simulink model "nuri3s_dob__model_free"  (R2024b)
settings: Solver=VariableStepAuto  StartTime=0.0  StopTime=5  RelTol=1e-3
undefined symbols (not defined in the file): q_goal_rad, q_start
libraries: robotmaniplib x1, robotcorelib x1, simulink_extras x1
settings Model: Creator=변재형  LastModifiedBy=변재형

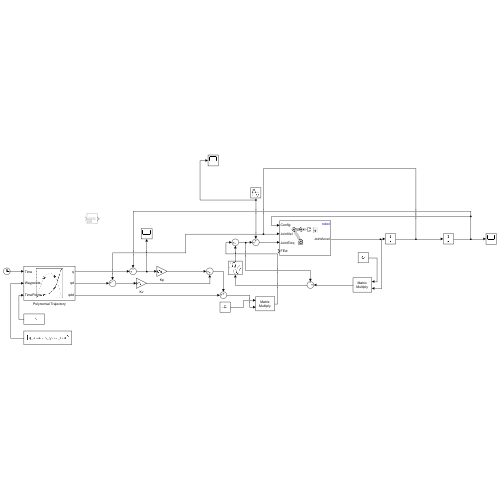
[thumbnail: Simulink's stored preview of the top-level diagram]
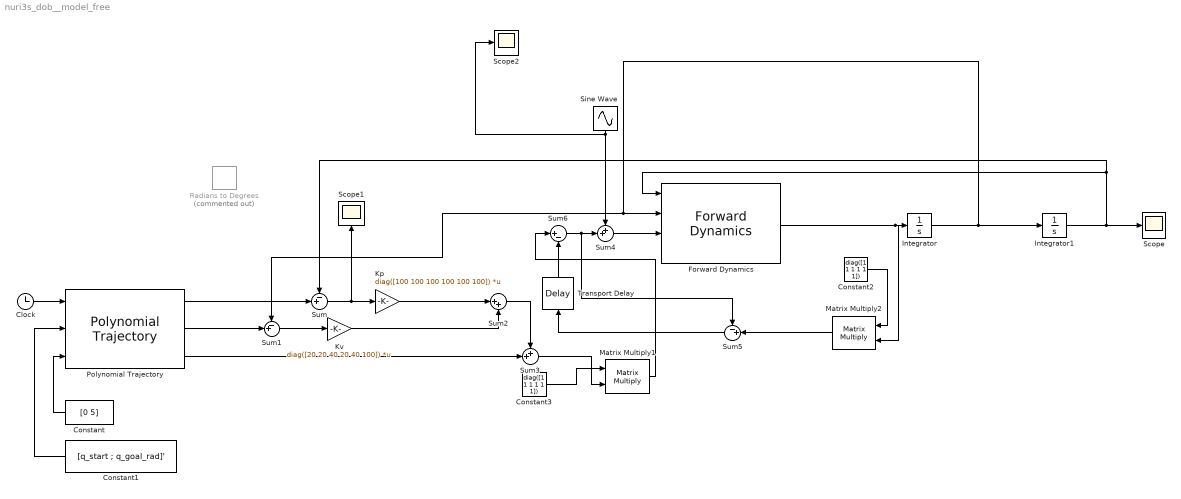
== system nuri3s_dob__model_free ==
  Clock : Clock
  Constant : Constant  Value=[0 5]
  Constant1 : Constant  Value=[q_start ; q_goal_rad]'
  Constant2 : Constant  Value=diag([1 1 1 1 1 1])
  Constant3 : Constant  Value=diag([1 1 1 1 1 1])
  Forward Dynamics : robotmaniplib/Forward Dynamics  RigidBodyTree=robot  SimulateUsing=Interpreted execution
  Integrator : Integrator
  Integrator1 : Integrator
  Kp : Gain  Gain=diag([100 100 100 100 100 100])  Multiplication=Matrix(K*u)
  Kv : Gain  Gain=diag([20 20 40 20 40 100])  Multiplication=Matrix(K*u)
  Matrix Multiply1 : Product  Multiplication=Matrix(*)
  Matrix Multiply2 : Product  Multiplication=Matrix(*)
  Polynomial Trajectory : robotcorelib/Polynomial Trajectory  WaypointSource=External  Waypoints=[ 0, 2, 1, 5, 0; -1, 3, 1, 4, 4 ]  TimePoints=[ 0, 1, 2, 3, 4 ]  TimeInterval=[ 1, 4 ]  Method=Quintic Polynomial  ParameterSource=Internal  VelocityBoundaryCondition=zeros( 6, 2 )  AccelerationBoundaryCondition=zeros( 6, 2 )  SimulateUsing=Interpreted execution
  Radians to Degrees : simulink_extras/Transformations/Radians to Degrees  Commented=on
  Scope : Scope
  Scope1 : Scope
  Scope2 : Scope
  Sine Wave : Sin  Amplitude=0.1  Frequency=10  SampleTime=0
  Sum : Sum  Inputs=-+|
  Sum1 : Sum  Inputs=-+|
  Sum2 : Sum  Inputs=|++
  Sum3 : Sum  Inputs=++|
  Sum4 : Sum  Inputs=++|
  Sum5 : Sum  Inputs=-+|
  Sum6 : Sum  Inputs=|+-
  Transport Delay : TransportDelay  DelayTime=0.001
  wires:
  Constant1/1 -> Polynomial Trajectory/2
  Constant/1 -> Polynomial Trajectory/3
  Clock/1 -> Polynomial Trajectory/1
  Forward Dynamics/1 -> Matrix Multiply2/2, Integrator/1
  Integrator/1 -> Sum1/1, Forward Dynamics/2, Integrator1/1
  Integrator1/1 -> Scope/1, Sum/1, Forward Dynamics/1
  Polynomial Trajectory/1 -> Sum/2
  Sum/1 -> Scope1/1, Kp/1
  Polynomial Trajectory/2 -> Sum1/2
  Sum1/1 -> Kv/1
  Kp/1 -> Sum2/1
  Kv/1 -> Sum2/2
  Polynomial Trajectory/3 -> Sum3/2
  Sum2/1 -> Sum3/1
  Sine Wave/1 -> Scope2/1, Sum4/1
  Sum4/1 -> Forward Dynamics/3
  Constant3/1 -> Matrix Multiply1/1
  Sum3/1 -> Matrix Multiply1/2
  Constant2/1 -> Matrix Multiply2/1
  Matrix Multiply2/1 -> Sum5/2
  Sum6/1 -> Sum5/1, Sum4/2
  Sum5/1 -> Transport Delay/1
  Transport Delay/1 -> Sum6/2
  Matrix Multiply1/1 -> Sum6/1
